simulink model "grid"  (R2025b)
settings: Solver=ode23t  StartTime=0.0  StopTime=0.1  RelTol=1e-3
InitFcn:
  | [P, Q, f_g, f_sw, V_dc, V_g, L_1, L_2, C_f, R_f] = lcl_param();
values from neighbouring files (symbols this model uses):
  f_g = 60    [lcl_param.m]
  f_sw = 5000    [Grid_connected_LCL_filter_code.m]    (also in LCL_filter_code.m; Load_connected_LCL_filter_code.m = 5040; Minor_Final_code.m; lcl_param.m = 15000)
  Q = 250    [lcl_param.m]
  R_f = 3*R_f    [lcl_param.m]
  V_dc = 400    [lcl_param.m]
  V_g = 120 * sqrt(3)    [lcl_param.m]
undefined symbols (not defined in the file or in its folder): PWMGenerator_2_Level__class, Three_PhaseProgrammableV_class, Three_PhaseV_IMeasuremen_class, UniversalBridge_class
libraries: fl_lib x22, nesl_utility x13, ee_lib x5, eeGeneralControl x3, slpidlib x3, eeTransforms x3, eePwmGeneratorTwoLevel x1, eeTotalHarmonicDistorsion x1, sps_lib x1
(part 1 of 2)
settings Model: Creator=swaya  LastModifiedBy=swaya
settings DebuggingCC: SaveWithParameterizedLinksMsg=none

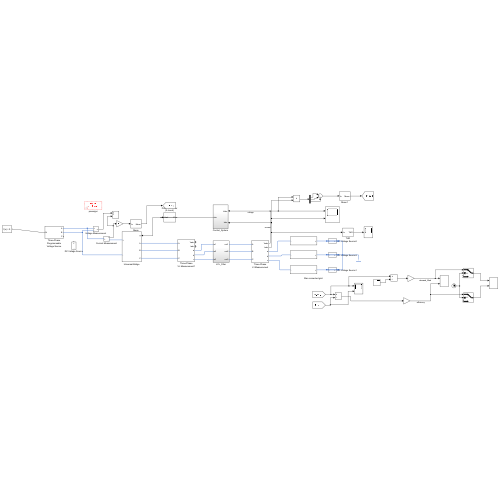
[thumbnail: Simulink's stored preview of the top-level diagram]
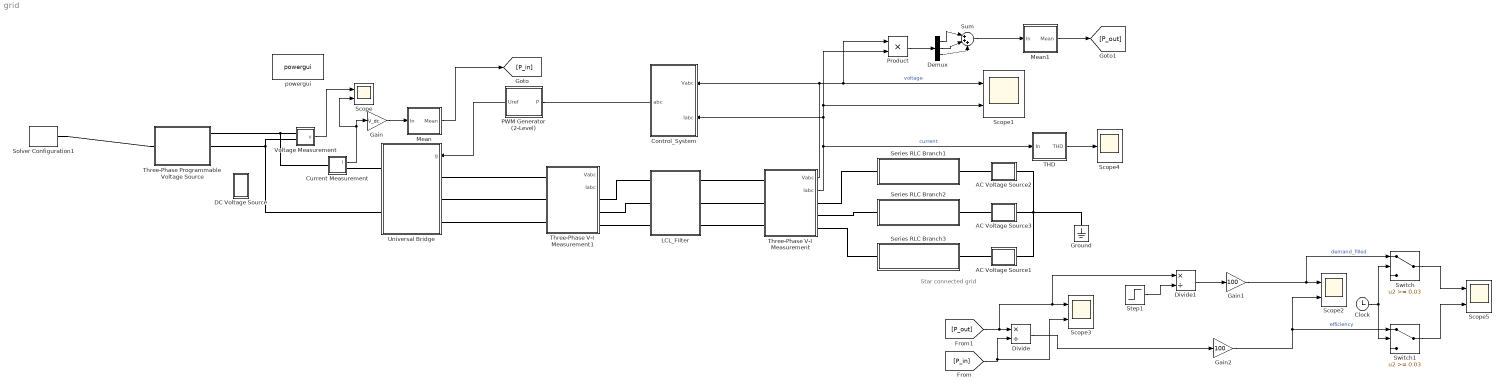
== system grid ==
  note: Star connected grid
  AC Voltage Source1 : Subsystem
      settings: OpenFcn=elec.conv.unmask(gcb);
  AC Voltage Source2 : Subsystem
      settings: OpenFcn=elec.conv.unmask(gcb);
  AC Voltage Source3 : Subsystem
      settings: OpenFcn=elec.conv.unmask(gcb);
  Clock : Clock
  Control_System : Subsystem
  Current Measurement : Subsystem
      settings: OpenFcn=elec.conv.unmask(gcb);
  DC Voltage Source : Subsystem
      settings: OpenFcn=elec.conv.unmask(gcb);
  Demux : Demux  Outputs=3
  Divide : Product  Inputs=*/
  Divide1 : Product  Inputs=*/
  Gain : Gain  Gain=V_dc
  Gain1 : Gain  Gain=100
  Gain2 : Gain  Gain=100
  Ground : fl_lib/Electrical/Electrical Elements/Electrical Reference
  LCL_Filter : Subsystem
  Mean : Subsystem
      settings: OpenFcn=elec.conv.unmask(gcb);
  Mean1 : Subsystem
      settings: OpenFcn=elec.conv.unmask(gcb);
  PWM Generator (2-Level) : Subsystem
      settings: OpenFcn=elec.conv.unmask(gcb);
  Product : Product
  Scope{,1..3,5} (5 alike) : Scope  NumInputPorts=2
      Scope settings: ActiveDisplayYMinimum=387.5  ActiveDisplayYMaximum=512.5
      Scope1 settings: ActiveDisplayYMinimum=-238.93464  ActiveDisplayYMaximum=235.18546  DataLoggingVariableName=ScopeData3
      Scope2 settings: ActiveDisplayYMinimum=-15.53558  ActiveDisplayYMaximum=139.82019  DataLoggingVariableName=ScopeData2
      Scope3 settings: ActiveDisplayYMinimum=-632.55835  ActiveDisplayYMaximum=5693.02515
      Scope5 settings: ActiveDisplayYMinimum=-12.69456  ActiveDisplayYMaximum=114.25108  DataLoggingVariableName=ScopeData4
  Scope4 : Scope
      settings: ActiveDisplayYMinimum=-0.05317  ActiveDisplayYMaximum=0.47849  DataLoggingVariableName=ScopeData3
  Series RLC Branch1 : Subsystem
      settings: OpenFcn=elec.conv.unmask(gcb);
  Series RLC Branch2 : Subsystem
      settings: OpenFcn=elec.conv.unmask(gcb);
  Series RLC Branch3 : Subsystem
      settings: OpenFcn=elec.conv.unmask(gcb);
  Solver Configuration1 : nesl_utility/Solver Configuration  PhysicalDomain=network_engine_domain  SubClassName=solver  LeftPortType=input  RightPortType=generic  Tones=[]  Harmonics=[]  SimulateNoise=off  Profile=off  UseLocalSampling=off  EnableSwitchedLinearOptims=on  FrequencyDomain=off  UseCCode=off  RelTol=0.001  AbsTol=0.001  MinStep=1e-09  ToWorkspace=off  RevertToSquareIcSolve=off  NumHomotopyIterations=100  PhasorMode=off  PhasorModeNumHarmonics=1  ConsistencySolver=NEWTON_XTOL_AFTER_FTOL  IndexReductionMethod=DerivativeReplacement  DoDC=off  ResidualTolerance=1e-09  ConsistencyTolSource=GLOBAL  ConsistencyAbsTol=0.001  ConsistencyRelTol=0.001  ConsistencyTolFactor=0.001  UseLocalSolver=off  LocalSolverChoice=NE_BACKWARD_EULER_ADVANCER  ResolveIndetEquations=on  FunctionEvalNumThread=1  LocalSolverSampleTime=0.001  DoFixedCost=off  MaxNonlinIter=3  MaxModeIter=2  ComputeImpulses=off  ImpulseIterations=2  LinearAlgebra=auto  LinearAlgebraNumThread=0  EquationFormulation=NE_TIME_EF  DelaysMemoryBudget=1024  AutomaticFiltering=on  FilteringTimeConstant=0.001  PartitionStorageMethod=AS_NEEDED  PartitionMemoryBudget=1024  PartitionMethod=ROBUST  MultibodyUseLocalSolver=off  MultibodyLocalSolverChoice=ODE1  MultibodyLocalSolverSampleTime=0.001
  Step1 : Step  Time=0.04  Before=3000  After=5000  SampleTime=0
  Sum : Sum  Inputs=|+++
  Switch : Switch  Threshold=0.03  SaturateOnIntegerOverflow=off  InputSameDT=off
  Switch1 : Switch  Threshold=0.03  SaturateOnIntegerOverflow=off  InputSameDT=off
  THD : Subsystem
      settings: OpenFcn=elec.conv.unmask(gcb);
  Three-Phase Programmable Voltage Source : Subsystem
      settings: OpenFcn=elec.conv.unmask(gcb);
  Three-Phase V-I Measurement : Subsystem
      settings: OpenFcn=elec.conv.unmask(gcb);
  Three-Phase V-I Measurement1 : Subsystem
      settings: OpenFcn=elec.conv.unmask(gcb);
  Universal Bridge : Subsystem
      settings: OpenFcn=elec.conv.unmask(gcb);
  Voltage Measurement : Subsystem
      settings: OpenFcn=elec.conv.unmask(gcb);
  powergui : sps_lib/powergui  Priority=1  SimulationMode=Discrete  SampleTime=50e-8  frequency=60  Iterations=50  frequencyindice=0  Pbase=100e6  ErrMax=1e-4  UnitsV=kV  UnitsW=MW  buscounter=0  FunctionMessages=off  echomessages=off  EnableUseOfTLC=off  CurrentSourceSwitches=off  DisableSnubberDevices=off  DisableRonSwitches=off  DisableVfSwitches=off  DisplayEquations=off  AutomaticDiscreteSolvers=off  SolverType=Tustin/Backward Euler (TBE)  Interpol=off  ExternalGateDelay=off  methode=off  Ts=100  x0status=blocks  SPID=on  SwTol=0  HookPort=off  NonlinearTolerance=1e-4  nMaxIteration=100  ContinueOnMaxIteration=off  RestoreLinks=warning  ResistiveCurrentMeasurement=off  Frange=[0:2:500]  Ylog=off  Xlog=on  ShowGrid=off  save=off  variable=ZData  structure=0  ZoomFFT=off  StartTime=0.0  cycles=1  DisplayStyle=1  fundamental=60  FreqAxis=off  MaxFrequency=1000  frequencyindicesteady=1  RmsSteady=1  display=off
  wires:
  PWM Generator (2-Level)/1(P) -> Universal Bridge/1(g)
  Three-Phase V-I Measurement/1(Vabc) -> Product/1, Scope1/1, Control_System/1(Vabc)  "voltage"
  Three-Phase V-I Measurement/2(Iabc) -> THD/1(In), Product/2, Scope1/2, Control_System/2(Iabc)  "current"
  Control_System/1(abc) -> PWM Generator (2-Level)/1(Uref)
  Product/1 -> Demux/1
  Demux/1 -> Sum/1
  Demux/2 -> Sum/2
  Demux/3 -> Sum/3
  Current Measurement/1(i) -> Scope/2, Gain/1
  THD/1(THD) -> Scope4/1
  Gain/1 -> Mean/1(In)
  [P_out] -> Divide1/1, Scope3/1, Divide/1
  [P_in] -> Scope3/2, Divide/2
  Divide1/1 -> Gain1/1
  Gain1/1 -> Switch/1, Scope2/1  "demand_filled"
  Mean/1(Mean) -> [P_in]
  Divide/1 -> Gain2/1
  Gain2/1 -> Switch1/1, Scope2/2  "efficiency"
  Sum/1 -> Mean1/1(In)
  Mean1/1(Mean) -> [P_out]
  Clock/1 -> Switch/2, Switch1/2
  Switch/1 -> Scope5/1
  Switch1/1 -> Scope5/2
  Step1/1 -> Divide1/2
  Voltage Measurement/1(v) -> Scope/1
  connections:
  LCL_Filter/RConn1 -- Three-Phase V-I Measurement/LConn1
  LCL_Filter/RConn2 -- Three-Phase V-I Measurement/LConn2
  LCL_Filter/RConn3 -- Three-Phase V-I Measurement/LConn3
  Three-Phase V-I Measurement1/LConn1 -- Universal Bridge/LConn1
  Three-Phase V-I Measurement1/LConn2 -- Universal Bridge/LConn2
  Three-Phase V-I Measurement1/LConn3 -- Universal Bridge/LConn3
  Three-Phase V-I Measurement1/RConn1 -- LCL_Filter/LConn1
  Three-Phase V-I Measurement1/RConn2 -- LCL_Filter/LConn2
  Three-Phase V-I Measurement1/RConn3 -- LCL_Filter/LConn3
  Series RLC Branch2/LConn1 -- AC Voltage Source3/RConn1
  AC Voltage Source2/RConn1 -- Series RLC Branch1/LConn1
  Series RLC Branch3/LConn1 -- AC Voltage Source1/RConn1
  AC Voltage Source2/LConn1 -- Ground/LConn1 -- AC Voltage Source1/LConn1 -- AC Voltage Source3/LConn1
  Three-Phase V-I Measurement/RConn1 -- Series RLC Branch1/RConn1
  Three-Phase V-I Measurement/RConn2 -- Series RLC Branch2/RConn1
  Three-Phase V-I Measurement/RConn3 -- Series RLC Branch3/RConn1
  Current Measurement/RConn1 -- Universal Bridge/RConn1
  Three-Phase Programmable Voltage Source/RConn1 -- Current Measurement/LConn1 -- Voltage Measurement/LConn1
  Three-Phase Programmable Voltage Source/RConn2 -- Voltage Measurement/LConn2 -- Universal Bridge/RConn2
  Solver Configuration1/RConn1 -- Three-Phase Programmable Voltage Source/LConn1

== system grid/AC Voltage Source1 ==
  AC Voltage Source : fl_lib/Electrical/Electrical Sources/AC Voltage Source  amp=V_g*sqrt(2/3) V  shift=120 deg  frequency=f_g Hz
  - : PMIOPort  Side=Left
  + : PMIOPort  Port=2  Side=Right
  connections:
  AC Voltage Source/LConn1 -- +/RConn1
  -/RConn1 -- AC Voltage Source/RConn1

== system grid/AC Voltage Source2 ==
  AC Voltage Source : fl_lib/Electrical/Electrical Sources/AC Voltage Source  amp=V_g*sqrt(2/3) V  shift=0 deg  frequency=f_g Hz
  - : PMIOPort  Side=Left
  + : PMIOPort  Port=2  Side=Right
  connections:
  AC Voltage Source/LConn1 -- +/RConn1
  -/RConn1 -- AC Voltage Source/RConn1

== system grid/AC Voltage Source3 ==
  AC Voltage Source : fl_lib/Electrical/Electrical Sources/AC Voltage Source  amp=V_g*sqrt(2/3) V  shift=-120 deg  frequency=f_g Hz
  - : PMIOPort  Side=Left
  + : PMIOPort  Port=2  Side=Right
  connections:
  AC Voltage Source/LConn1 -- +/RConn1
  -/RConn1 -- AC Voltage Source/RConn1

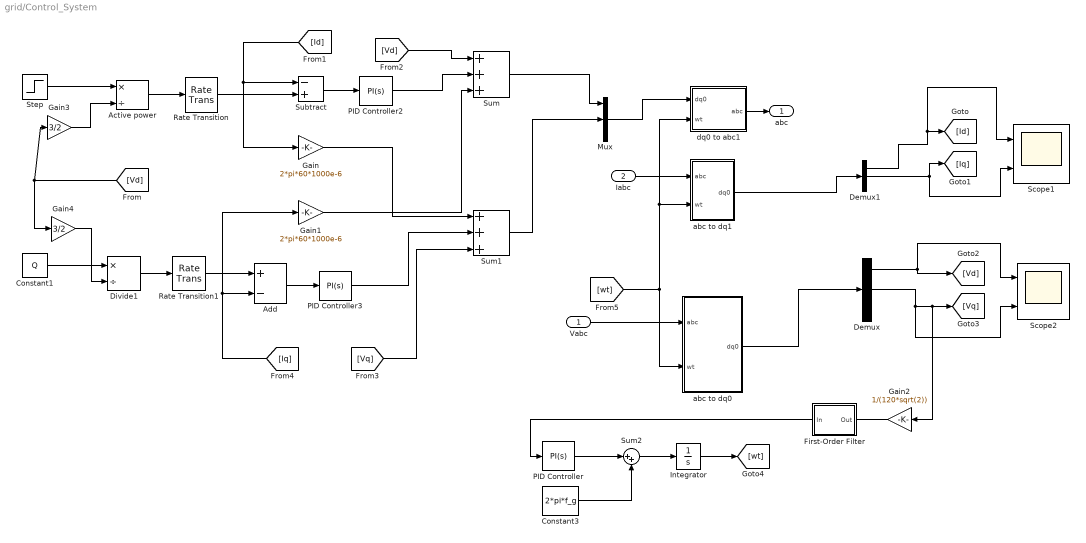
== system grid/Control_System ==
  Vabc : Inport
  Iabc : Inport  Port=2
  Active power : Product  Inputs=*/
  Add : Sum  Inputs=+-
  Constant1 : Constant  Value=Q
  Constant3 : Constant  Value=2*pi*f_g
  Demux : Demux  Outputs=3
  Demux1 : Demux  Outputs=3
  Divide1 : Product  Inputs=*/
  First-Order Filter : Subsystem
      settings: OpenFcn=elec.conv.unmask(gcb);
  Gain : Gain  Gain=2*pi*60*1000e-6
  Gain1 : Gain  Gain=2*pi*60*1000e-6
  Gain2 : Gain  Gain=1/(120*sqrt(2))
  Gain3 : Gain  Gain=3/2
  Gain4 : Gain  Gain=3/2
  Integrator : Integrator
  Mux : Mux  Inputs=3
  PID Controller : slpidlib/PID Controller  Controller=PI  Form=Parallel  TimeDomain=Continuous-time  UseExternalTs=off  SampleTime=-1  IntegratorMethod=Forward Euler  FilterMethod=Forward Euler  ControllerParametersSource=internal  P=-0.26  I=-5.8  UseKiTs=off  D=10  UseExternalDerivativeSource=off  N=100  UseFilter=on  TunerSelectOption=Transfer Function Based (PID Tuner App)  InitialConditionSource=internal  InitialConditionForIntegrator=0  InitialConditionForFilter=0  DifferentiatorICPrevScaledInput=0  ExternalReset=none  TrackingMode=off  Kt=1  LimitOutput=on  SatLimitsSource=internal  UpperSaturationLimit=inf  LowerSaturationLimit=-inf  LinearizeAsGain=on  AntiWindupMode=back-calculation  Kb=1  LimitIntegrator=off  UpperIntegratorSaturationLimit=100  LowerIntegratorSaturationLimit=-inf  POutMin=[]  POutMax=[]  IOutMin=[]  IOutMax=[]  DOutMin=[]  DOutMax=[]  NOutMin=[]  NOutMax=[]  SumOutMin=[]  SumOutMax=[]  SaturationOutMin=[]  SaturationOutMax=[]  PParamMin=[]  PParamMax=[]  IParamMin=[]  IParamMax=[]  DParamMin=[]  DParamMax=[]  NParamMin=[]  NParamMax=[]  KbParamMin=[]  KbParamMax=[]  KtParamMin=[]  KtParamMax=[]  KbOutMin=[]  KbOutMax=[]  KtOutMin=[]  KtOutMax=[]  IntegratorOutMin=[]  IntegratorOutMax=[]  FilterOutMin=[]  FilterOutMax=[]  SumI1OutMin=[]  SumI1OutMax=[]  SumI2OutMin=[]  SumI2OutMax=[]  SumI3OutMin=[]  SumI3OutMax=[]  SumI4OutMin=[]  SumI4OutMax=[]  SumDOutMin=[]  SumDOutMax=[]  DifferentiatorOutMin=[]  DifferentiatorOutMax=[]  FilterDiffOutCoefMin=[]  FilterDiffOutCoefMax=[]  ReciprocalOutMin=[]  ReciprocalOutMax=[]  SumDenOutMin=[]  SumDenOutMax=[]  SumNumOutMin=[]  SumNumOutMax=[]  DivideOutMin=[]  DivideOutMax=[]  UdiffTsProdOutMin=[]  UdiffTsProdOutMax=[]  NTsProdOutMin=[]  NTsProdOutMax=[]  UintegralTsProdOutMin=[]  UintegralTsProdOutMax=[]  UngainTsProdOutMin=[]  UngainTsProdOutMax=[]  ClampingZeroOutDataTypeStr=Inherit: Inherit via back propagation  ClampingZeroOutMin=[]  ClampingZeroOutMax=[]  FilterDenConstantOutDataTypeStr=Inherit: Inherit via back propagation  FilterDenConstantOutMin=[]  FilterDenConstantOutMax=[]  PCopyOutDataTypeStr=Inherit: Inherit via back propagation  PCopyOutMin=[]  PCopyOutMax=[]  NCopyOutDataTypeStr=Inherit: Inherit via back propagation  NCopyOutMin=[]  NCopyOutMax=[]  IntegratorContinuousStateAttributes=''  IntegratorStateMustResolveToSignalObject=off  IntegratorRTWStateStorageClass=Auto  FilterContinuousStateAttributes=''  FilterStateMustResolveToSignalObject=off  FilterRTWStateStorageClass=Auto  ParallelPVariant=InternalParameters  IdealPVariant=Disabled  IVariant=InternalParameters  DVariant=Disabled  IntegratorVariant=Continuous  SatVariant=Enabled  AWVariant=BackCalculation  PCopyVariant=Disabled  TRVariant=Disabled  FdbkBlocksVariant=Forward  IdealPFdbkVariant=Disabled  SatFdbkVariant=Disabled  DerivativeFilterVariant=Disabled  NVariant=Disabled  NCopyVariant=Disabled_SignalSpec  FilterICVariant=Disabled  IntegratorICVariant=InternalICs  ExternalResetVariant=Disabled  TRSumVariant=Passthrough  SumFdbkVariant=Disabled  SumVariant=Sum_PI  TsampFilterVariant=InternalTs  TsampNgainVariant=Passthrough  TsampIntegralVariant=Disabled_SignalSpec  ExternalSaturationOutDataTypeStr=Inherit: Same as second input  DerivativeSourceVariant=Disabled  PreIntVariant=InternalPreInt
  PID Controller2 : slpidlib/PID Controller  Controller=PI  Form=Parallel  TimeDomain=Continuous-time  UseExternalTs=off  SampleTime=-1  IntegratorMethod=Forward Euler  FilterMethod=Forward Euler  ControllerParametersSource=internal  P=5  I=5000  UseKiTs=off  D=5  UseExternalDerivativeSource=off  N=100  UseFilter=on  TunerSelectOption=Transfer Function Based (PID Tuner App)  InitialConditionSource=internal  InitialConditionForIntegrator=0  InitialConditionForFilter=0  DifferentiatorICPrevScaledInput=0  ExternalReset=none  TrackingMode=off  Kt=1  LimitOutput=on  SatLimitsSource=internal  UpperSaturationLimit=inf  LowerSaturationLimit=-inf  LinearizeAsGain=on  AntiWindupMode=back-calculation  Kb=1  LimitIntegrator=off  UpperIntegratorSaturationLimit=inf  LowerIntegratorSaturationLimit=-inf  POutMin=[]  POutMax=[]  IOutMin=[]  IOutMax=[]  DOutMin=[]  DOutMax=[]  NOutMin=[]  NOutMax=[]  SumOutMin=[]  SumOutMax=[]  SaturationOutMin=[]  SaturationOutMax=[]  PParamMin=[]  PParamMax=[]  IParamMin=[]  IParamMax=[]  DParamMin=[]  DParamMax=[]  NParamMin=[]  NParamMax=[]  KbParamMin=[]  KbParamMax=[]  KtParamMin=[]  KtParamMax=[]  KbOutMin=[]  KbOutMax=[]  KtOutMin=[]  KtOutMax=[]  IntegratorOutMin=[]  IntegratorOutMax=[]  FilterOutMin=[]  FilterOutMax=[]  SumI1OutMin=[]  SumI1OutMax=[]  SumI2OutMin=[]  SumI2OutMax=[]  SumI3OutMin=[]  SumI3OutMax=[]  SumI4OutMin=[]  SumI4OutMax=[]  SumDOutMin=[]  SumDOutMax=[]  DifferentiatorOutMin=[]  DifferentiatorOutMax=[]  FilterDiffOutCoefMin=[]  FilterDiffOutCoefMax=[]  ReciprocalOutMin=[]  ReciprocalOutMax=[]  SumDenOutMin=[]  SumDenOutMax=[]  SumNumOutMin=[]  SumNumOutMax=[]  DivideOutMin=[]  DivideOutMax=[]  UdiffTsProdOutMin=[]  UdiffTsProdOutMax=[]  NTsProdOutMin=[]  NTsProdOutMax=[]  UintegralTsProdOutMin=[]  UintegralTsProdOutMax=[]  UngainTsProdOutMin=[]  UngainTsProdOutMax=[]  ClampingZeroOutDataTypeStr=Inherit: Inherit via back propagation  ClampingZeroOutMin=[]  ClampingZeroOutMax=[]  FilterDenConstantOutDataTypeStr=Inherit: Inherit via back propagation  FilterDenConstantOutMin=[]  FilterDenConstantOutMax=[]  PCopyOutDataTypeStr=Inherit: Inherit via back propagation  PCopyOutMin=[]  PCopyOutMax=[]  NCopyOutDataTypeStr=Inherit: Inherit via back propagation  NCopyOutMin=[]  NCopyOutMax=[]  IntegratorContinuousStateAttributes=''  IntegratorStateMustResolveToSignalObject=off  IntegratorRTWStateStorageClass=Auto  FilterContinuousStateAttributes=''  FilterStateMustResolveToSignalObject=off  FilterRTWStateStorageClass=Auto  ParallelPVariant=InternalParameters  IdealPVariant=Disabled  IVariant=InternalParameters  DVariant=Disabled  IntegratorVariant=Continuous  SatVariant=Enabled  AWVariant=BackCalculation  PCopyVariant=Disabled  TRVariant=Disabled  FdbkBlocksVariant=Forward  IdealPFdbkVariant=Disabled  SatFdbkVariant=Disabled  DerivativeFilterVariant=Disabled  NVariant=Disabled  NCopyVariant=Disabled_SignalSpec  FilterICVariant=Disabled  IntegratorICVariant=InternalICs  ExternalResetVariant=Disabled  TRSumVariant=Passthrough  SumFdbkVariant=Disabled  SumVariant=Sum_PI  TsampFilterVariant=InternalTs  TsampNgainVariant=Passthrough  TsampIntegralVariant=Disabled_SignalSpec  ExternalSaturationOutDataTypeStr=Inherit: Same as second input  DerivativeSourceVariant=Disabled  PreIntVariant=InternalPreInt
  PID Controller3 : slpidlib/PID Controller  Controller=PI  Form=Parallel  TimeDomain=Continuous-time  UseExternalTs=off  SampleTime=-1  IntegratorMethod=Forward Euler  FilterMethod=Forward Euler  ControllerParametersSource=internal  P=5  I=5000  UseKiTs=off  D=5  UseExternalDerivativeSource=off  N=100  UseFilter=on  TunerSelectOption=Transfer Function Based (PID Tuner App)  InitialConditionSource=internal  InitialConditionForIntegrator=0  InitialConditionForFilter=0  DifferentiatorICPrevScaledInput=0  ExternalReset=none  TrackingMode=off  Kt=1  LimitOutput=on  SatLimitsSource=internal  UpperSaturationLimit=inf  LowerSaturationLimit=-inf  LinearizeAsGain=on  AntiWindupMode=back-calculation  Kb=1  LimitIntegrator=off  UpperIntegratorSaturationLimit=inf  LowerIntegratorSaturationLimit=-inf  POutMin=[]  POutMax=[]  IOutMin=[]  IOutMax=[]  DOutMin=[]  DOutMax=[]  NOutMin=[]  NOutMax=[]  SumOutMin=[]  SumOutMax=[]  SaturationOutMin=[]  SaturationOutMax=[]  PParamMin=[]  PParamMax=[]  IParamMin=[]  IParamMax=[]  DParamMin=[]  DParamMax=[]  NParamMin=[]  NParamMax=[]  KbParamMin=[]  KbParamMax=[]  KtParamMin=[]  KtParamMax=[]  KbOutMin=[]  KbOutMax=[]  KtOutMin=[]  KtOutMax=[]  IntegratorOutMin=[]  IntegratorOutMax=[]  FilterOutMin=[]  FilterOutMax=[]  SumI1OutMin=[]  SumI1OutMax=[]  SumI2OutMin=[]  SumI2OutMax=[]  SumI3OutMin=[]  SumI3OutMax=[]  SumI4OutMin=[]  SumI4OutMax=[]  SumDOutMin=[]  SumDOutMax=[]  DifferentiatorOutMin=[]  DifferentiatorOutMax=[]  FilterDiffOutCoefMin=[]  FilterDiffOutCoefMax=[]  ReciprocalOutMin=[]  ReciprocalOutMax=[]  SumDenOutMin=[]  SumDenOutMax=[]  SumNumOutMin=[]  SumNumOutMax=[]  DivideOutMin=[]  DivideOutMax=[]  UdiffTsProdOutMin=[]  UdiffTsProdOutMax=[]  NTsProdOutMin=[]  NTsProdOutMax=[]  UintegralTsProdOutMin=[]  UintegralTsProdOutMax=[]  UngainTsProdOutMin=[]  UngainTsProdOutMax=[]  ClampingZeroOutDataTypeStr=Inherit: Inherit via back propagation  ClampingZeroOutMin=[]  ClampingZeroOutMax=[]  FilterDenConstantOutDataTypeStr=Inherit: Inherit via back propagation  FilterDenConstantOutMin=[]  FilterDenConstantOutMax=[]  PCopyOutDataTypeStr=Inherit: Inherit via back propagation  PCopyOutMin=[]  PCopyOutMax=[]  NCopyOutDataTypeStr=Inherit: Inherit via back propagation  NCopyOutMin=[]  NCopyOutMax=[]  IntegratorContinuousStateAttributes=''  IntegratorStateMustResolveToSignalObject=off  IntegratorRTWStateStorageClass=Auto  FilterContinuousStateAttributes=''  FilterStateMustResolveToSignalObject=off  FilterRTWStateStorageClass=Auto  ParallelPVariant=InternalParameters  IdealPVariant=Disabled  IVariant=InternalParameters  DVariant=Disabled  IntegratorVariant=Continuous  SatVariant=Enabled  AWVariant=BackCalculation  PCopyVariant=Disabled  TRVariant=Disabled  FdbkBlocksVariant=Forward  IdealPFdbkVariant=Disabled  SatFdbkVariant=Disabled  DerivativeFilterVariant=Disabled  NVariant=Disabled  NCopyVariant=Disabled_SignalSpec  FilterICVariant=Disabled  IntegratorICVariant=InternalICs  ExternalResetVariant=Disabled  TRSumVariant=Passthrough  SumFdbkVariant=Disabled  SumVariant=Sum_PI  TsampFilterVariant=InternalTs  TsampNgainVariant=Passthrough  TsampIntegralVariant=Disabled_SignalSpec  ExternalSaturationOutDataTypeStr=Inherit: Same as second input  DerivativeSourceVariant=Disabled  PreIntVariant=InternalPreInt
  Rate Transition : RateTransition  OutPortSampleTimeOpt=Inherit
  Rate Transition1 : RateTransition  OutPortSampleTimeOpt=Inherit
  Scope1 : Scope  NumInputPorts=2
      settings: ActiveDisplayYMinimum=-14.64317  ActiveDisplayYMaximum=37.77239
  Scope2 : Scope  NumInputPorts=2
      settings: ActiveDisplayYMinimum=165.62316  ActiveDisplayYMaximum=206.32488  DataLoggingVariableName=ScopeData2
  Step : Step  Time=0.04  Before=3000  After=5000  SampleTime=0
  Subtract : Sum  Inputs=-+
  Sum : Sum  Inputs=+++
  Sum1 : Sum  Inputs=+++
  Sum2 : Sum  Inputs=|++
  abc to dq0 : Subsystem
      settings: OpenFcn=elec.conv.unmask(gcb);
  abc to dq1 : Subsystem
      settings: OpenFcn=elec.conv.unmask(gcb);
  dq0 to abc1 : Subsystem
      settings: OpenFcn=elec.conv.unmask(gcb);
  abc : Outport
  wires:
  Demux1/1 -> [Id], Scope1/1
  [Iq] -> Gain1/1, Add/2
  [Vq] -> Sum1/3
  abc to dq1/1(dq0) -> Demux1/1
  Active power/1 -> Rate Transition/1
  dq0 to abc1/1(abc) -> abc/1
  Gain1/1 -> Sum/3
  [Vd] -> Sum/1
  abc to dq0/1(dq0) -> Demux/1
  [Id] -> Gain/1, Subtract/1
  Constant1/1 -> Divide1/1
  Demux/1 -> [Vd], Scope2/1
  Demux1/2 -> Scope1/2, [Iq]
  Mux/1 -> dq0 to abc1/1(dq0)
  Gain/1 -> Sum1/1
  Iabc/1 -> abc to dq1/1(abc)
  Vabc/1 -> abc to dq0/1(abc)
  Sum/1 -> Mux/1
  Sum1/1 -> Mux/2
  Rate Transition/1 -> Subtract/2
  Divide1/1 -> Rate Transition1/1
  Subtract/1 -> PID Controller2/1
  Add/1 -> PID Controller3/1
  PID Controller2/1 -> Sum/2
  PID Controller3/1 -> Sum1/2
  [wt] -> abc to dq0/2(wt), abc to dq1/2(wt), dq0 to abc1/2(wt)
  Demux/2 -> Scope2/2, Gain2/1, [Vq]
  Constant3/1 -> Sum2/2
  PID Controller/1 -> Sum2/1
  Integrator/1 -> [wt]
  First-Order Filter/1(Out) -> PID Controller/1
  Sum2/1 -> Integrator/1
  Gain2/1 -> First-Order Filter/1(In)
  Rate Transition1/1 -> Add/1
  [Vd] -> Gain4/1, Gain3/1
  Gain3/1 -> Active power/2
  Gain4/1 -> Divide1/2
  Step/1 -> Active power/1

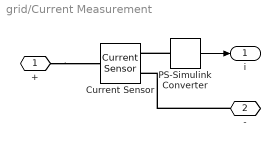
== system grid/Current Measurement ==
  Current Sensor : fl_lib/Electrical/Electrical Sensors/Current Sensor
  PS-Simulink Converter : nesl_utility/PS-Simulink Converter  PhysicalDomain=network_engine_domain  SubClassName=ps_output  LeftPortType=input  RightPortType=output  PseudoPeriodic=off  Frequencies=[]  VectorFormat=1-D array  Unit=A  AffineConversion=off
  + : PMIOPort  Side=Left
  - : PMIOPort  Port=2  Side=Right
  i : Outport  VectorParamsAs1DForOutWhenUnconnected=off
  wires:
  PS-Simulink Converter/1 -> i/1
  connections:
  +/RConn1 -- Current Sensor/LConn1
  -/RConn1 -- Current Sensor/RConn2
  PS-Simulink Converter/LConn1 -- Current Sensor/RConn1

== system grid/DC Voltage Source ==
  DC Voltage Source : fl_lib/Electrical/Electrical Sources/DC Voltage Source  v0=500 V
  - : PMIOPort  Side=Left
  + : PMIOPort  Port=2  Side=Right
  connections:
  DC Voltage Source/RConn1 -- -/RConn1
  DC Voltage Source/LConn1 -- +/RConn1

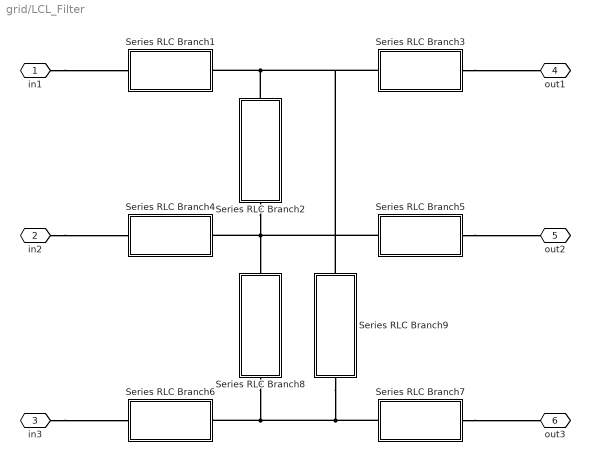
== system grid/LCL_Filter ==
  Series RLC Branch1 : Subsystem
      settings: OpenFcn=elec.conv.unmask(gcb);
  Series RLC Branch2 : Subsystem
      settings: OpenFcn=elec.conv.unmask(gcb);
  Series RLC Branch3 : Subsystem
      settings: OpenFcn=elec.conv.unmask(gcb);
  Series RLC Branch4 : Subsystem
      settings: OpenFcn=elec.conv.unmask(gcb);
  Series RLC Branch5 : Subsystem
      settings: OpenFcn=elec.conv.unmask(gcb);
  Series RLC Branch6 : Subsystem
      settings: OpenFcn=elec.conv.unmask(gcb);
  Series RLC Branch7 : Subsystem
      settings: OpenFcn=elec.conv.unmask(gcb);
  Series RLC Branch8 : Subsystem
      settings: OpenFcn=elec.conv.unmask(gcb);
  Series RLC Branch9 : Subsystem
      settings: OpenFcn=elec.conv.unmask(gcb);
  in1 : PMIOPort  Side=Left
  in2 : PMIOPort  Port=2  Side=Left
  in3 : PMIOPort  Port=3  Side=Left
  out1 : PMIOPort  Port=4  Side=Right
  out2 : PMIOPort  Port=5  Side=Right
  out3 : PMIOPort  Port=6  Side=Right
  connections:
  Series RLC Branch3/LConn1 -- out1/RConn1
  Series RLC Branch2/LConn1 -- Series RLC Branch3/RConn1 -- Series RLC Branch9/LConn1 -- Series RLC Branch1/LConn1
  in1/RConn1 -- Series RLC Branch1/RConn1
  Series RLC Branch5/RConn1 -- Series RLC Branch4/LConn1 -- Series RLC Branch8/LConn1 -- Series RLC Branch2/RConn1
  in2/RConn1 -- Series RLC Branch4/RConn1
  Series RLC Branch5/LConn1 -- out2/RConn1
  Series RLC Branch7/RConn1 -- Series RLC Branch9/RConn1 -- Series RLC Branch6/LConn1 -- Series RLC Branch8/RConn1
  Series RLC Branch7/LConn1 -- out3/RConn1
  in3/RConn1 -- Series RLC Branch6/RConn1

== system grid/Mean ==
  In : Inport
  Moving Average : eeGeneralControl/Moving Average  VariantControl=Variant1  LabelModeActiveChoice=Discrete  f=60  x0=0  BufferSize=8192  Ts=0
  Mean : Outport  VectorParamsAs1DForOutWhenUnconnected=off
  wires:
  Moving Average/1 -> Mean/1
  In/1 -> Moving Average/1

== system grid/Mean1 ==
  In : Inport
  Moving Average : eeGeneralControl/Moving Average  VariantControl=Variant1  LabelModeActiveChoice=Discrete  f=60  x0=0  BufferSize=8192  Ts=0
  Mean : Outport  VectorParamsAs1DForOutWhenUnconnected=off
  wires:
  Moving Average/1 -> Mean/1
  In/1 -> Moving Average/1

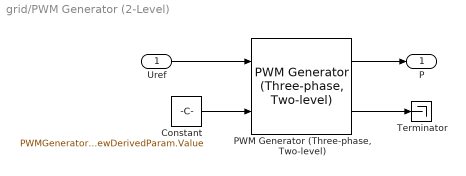
== system grid/PWM Generator (2-Level) ==
  Uref : Inport  SampleTime=PWMGenerator_2_Level__class([-1 1],0,60,f_sw,0,'Three-phase bridge (6 pulses)',0,'Natural').objParamMappingDerived.NewDerivedParam.SampleTime
  Constant : Constant  Value=PWMGenerator_2_Level__class([-1 1],0,60,f_sw,0,'Three-phase bridge (6 pulses)',0,'Natural').objParamMappingDerived.NewDerivedParam.Value  SampleTime=PWMGenerator_2_Level__class([-1 1],0,60,f_sw,0,'Three-phase bridge (6 pulses)',0,'Natural').objParamMappingDerived.NewDerivedParam.SampleTime
  "PWM Generator (Three-phase, Two-level)" : eePwmGeneratorTwoLevel/PWM Generator (Three-phase, Two-level)  PWMMode=Continuous PWM (CPWM)  CPWMMode=SPWM: sinusoidal PWM  DPWMMode=60 DPWM: 60 degree discontinuous PWM  fsw=f_sw  Ts=PWMGenerator_2_Level__class([-1 1],0,60,f_sw,0,'Three-phase bridge (6 pulses)',0,'Natural').objParamMappingDerived.NewDerivedParam.SampleTime
  Terminator : Terminator
  P : Outport  SampleTime=PWMGenerator_2_Level__class([-1 1],0,60,f_sw,0,'Three-phase bridge (6 pulses)',0,'Natural').objParamMappingDerived.NewDerivedParam.SampleTime  VectorParamsAs1DForOutWhenUnconnected=off
  wires:
  "PWM Generator (Three-phase, Two-level)"/2 -> Terminator/1
  "PWM Generator (Three-phase, Two-level)"/1 -> P/1
  Constant/1 -> "PWM Generator (Three-phase, Two-level)"/2
  Uref/1 -> "PWM Generator (Three-phase, Two-level)"/1

== system grid/Series RLC Branch1 ==
  Resistor : fl_lib/Electrical/Electrical Elements/Resistor  R=1 Ohm  i_specify=off  i_priority=None  i=0 A  i_nominal_specify=off  i_nominal_value=1  i_nominal_unit=A  v_specify=off  v_priority=None  v=0 V  v_nominal_specify=off  v_nominal_value=1  v_nominal_unit=V
  + : PMIOPort  Side=Left
  - : PMIOPort  Port=2  Side=Right
  connections:
  +/RConn1 -- Resistor/LConn1
  -/RConn1 -- Resistor/RConn1

== system grid/Series RLC Branch2 ==
  Resistor : fl_lib/Electrical/Electrical Elements/Resistor  R=1 Ohm  i_specify=off  i_priority=None  i=0 A  i_nominal_specify=off  i_nominal_value=1  i_nominal_unit=A  v_specify=off  v_priority=None  v=0 V  v_nominal_specify=off  v_nominal_value=1  v_nominal_unit=V
  + : PMIOPort  Side=Left
  - : PMIOPort  Port=2  Side=Right
  connections:
  +/RConn1 -- Resistor/LConn1
  -/RConn1 -- Resistor/RConn1

== system grid/Series RLC Branch3 ==
  Resistor : fl_lib/Electrical/Electrical Elements/Resistor  R=1 Ohm  i_specify=off  i_priority=None  i=0 A  i_nominal_specify=off  i_nominal_value=1  i_nominal_unit=A  v_specify=off  v_priority=None  v=0 V  v_nominal_specify=off  v_nominal_value=1  v_nominal_unit=V
  + : PMIOPort  Side=Left
  - : PMIOPort  Port=2  Side=Right
  connections:
  +/RConn1 -- Resistor/LConn1
  -/RConn1 -- Resistor/RConn1

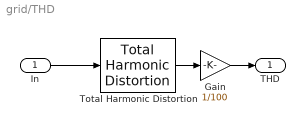
== system grid/THD ==
  In : Inport
  Gain : Gain  Gain=1/100  SampleTime=0
  Total Harmonic Distortion : eeTotalHarmonicDistorsion/Total Harmonic Distortion  f=f_g  Ts=0
  THD : Outport  VectorParamsAs1DForOutWhenUnconnected=off
  wires:
  Gain/1 -> THD/1
  In/1 -> Total Harmonic Distortion/1
  Total Harmonic Distortion/1 -> Gain/1

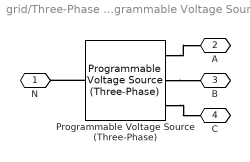
== system grid/Three-Phase Programmable Voltage Source ==
  Programmable Voltage Source (Three-Phase) : ee_lib/Sources/Programmable Voltage Source (Three-Phase)  magnitude_type=3  vline_rms=565.6854 V  magn_ramp=Three_PhaseProgrammableV_class([565.685424949238 0 0],0.25,10,0.3,[3 0.2 -25 0],[2 0.15 35 2]).objParamMappingDerived.NewDerivedParam.magn_ramp V/s  magn_step=Three_PhaseProgrammableV_class([565.685424949238 0 0],0.25,10,0.3,[3 0.2 -25 0],[2 0.15 35 2]).objParamMappingDerived.NewDerivedParam.magn_step V  magn_modu_magn=Three_PhaseProgrammableV_class([565.685424949238 0 0],0.25,10,0.3,[3 0.2 -25 0],[2 0.15 35 2]).objParamMappingDerived.NewDerivedParam.magn_modu_magn V  magn_modu_freq=2 Hz  magn_t1=0.08 s  magn_t2=0.2 s  frequency_type=1  freq=0 Hz  freq_ramp=10 Hz/s  freq_step=0.25 Hz  freq_modu_magn=0.3 Hz  freq_modu_freq=2 Hz  freq_t1=0.08 s  freq_t2=0.2 s  phase_type=1  shift=0 deg  phase_ramp=10 deg/s  phase_step=0.25 deg  phase_modu_magn=0.3 deg  phase_modu_freq=2 Hz  phase_t1=0.08 s  phase_t2=0.2 s  impedance_option=0  SShortCircuit=1e6 V*A  XR=15  R=0.01 Ohm  L=3.97e-4 H  G_parasitic=0 1/Ohm  harmonic_option=0  harmonic_orders=Three_PhaseProgrammableV_class([565.685424949238 0 0],0.25,10,0.3,[3 0.2 -25 0],[2 0.15 35 2]).objParamMappingDerived.NewDerivedParam.harmonic_orders  harmonic_ratios=Three_PhaseProgrammableV_class([565.685424949238 0 0],0.25,10,0.3,[3 0.2 -25 0],[2 0.15 35 2]).objParamMappingDerived.NewDerivedParam.harmonic_ratios  harmonic_shifts=Three_PhaseProgrammableV_class([565.685424949238 0 0],0.25,10,0.3,[3 0.2 -25 0],[2 0.15 35 2]).objParamMappingDerived.NewDerivedParam.harmonic_shifts deg  harmonic_sequences=Three_PhaseProgrammableV_class([565.685424949238 0 0],0.25,10,0.3,[3 0.2 -25 0],[2 0.15 35 2]).objParamMappingDerived.NewDerivedParam.harmonic_sequences  harmonic_t1=0.05 s  harmonic_t2=3 s  I_specify=off  I_priority=None  I=[ 0 0 0 ] A  I_nominal_specify=off  I_nominal_value=1  I_nominal_unit=A  V_specify=off  V_priority=None  V=[ 0 0 0 ] V  V_nominal_specify=off  V_nominal_value=1  V_nominal_unit=V
      settings: InternalSimscapePortConfiguration="{\"Bottom\":[],\"Left\":[{\"id\":\"n\",\"label\":\"n\",\"type\":\"foundation.electrical.electrical\"}],\"Right\":[{\"id\":\"a\",\"label\":\"a\",\"type\":\"foundation.electrical.electrical\"},{\"id\":\"b\",\"label\":\"b\",\"type\":\"foundation.electrical.electrical\"},{\"id\":\"c\",\"label\":\"c\",\"type\":\"foundation.electrical.electrical\"}],\"Top\":[]}"
  N : PMIOPort  Side=Left
  A : PMIOPort  Port=2  Side=Right
  B : PMIOPort  Port=3  Side=Right
  C : PMIOPort  Port=4  Side=Right
  connections:
  Programmable Voltage Source (Three-Phase)/RConn2 -- B/RConn1
  Programmable Voltage Source (Three-Phase)/LConn1 -- N/RConn1
  Programmable Voltage Source (Three-Phase)/RConn3 -- C/RConn1
  Programmable Voltage Source (Three-Phase)/RConn1 -- A/RConn1

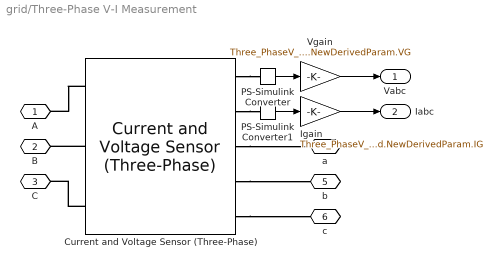
== system grid/Three-Phase V-I Measurement ==
  Current and Voltage Sensor (Three-Phase) : ee_lib/Sensors & Transducers/Current and Voltage Sensor (Three-Phase)  vMeasurementType=2  outputUnit=2  SRated=100000000 V*A  VRated=500000 V  I_specify=off  I_priority=None  I=[ 0 0 0 ] A  I_nominal_specify=off  I_nominal_value=1  I_nominal_unit=A  V_specify=off  V_priority=None  V=[ 0 0 0 ] V  V_nominal_specify=off  V_nominal_value=1  V_nominal_unit=V
      settings: InternalSimscapePortConfiguration="{\"Bottom\":[],\"Left\":[{\"id\":\"a1\",\"label\":\"a1\",\"type\":\"foundation.electrical.electrical\"},{\"id\":\"b1\",\"label\":\"b1\",\"type\":\"foundation.electrical.electrical\"},{\"id\":\"c1\",\"label\":\"c1\",\"type\":\"foundation.electrical.electrical\"}],\"Right\":[{\"id\":\"V_output\",\"label\":\"V\",\"type\":\"output\"},{\"id\":\"I_output\",\"label\":\"I\",\"type\":\"output\"},{\"id\":\"a2\",\"label\":\"a2\",\"type\":\"foundation.electrical.electrical\"},{\"id\":\"b2\",\"label\":\"b2\",\"type\":\"foundation.electrical.electrical\"},{\"id\":\"c2\",\"label\":\"c2\",\"type\":\"foundation.electrical.electrical\"}],\"Top\":[]}"
  Igain : Gain  Gain=Three_PhaseV_IMeasuremen_class('phase-to-ground','yes','off','off','off',100000000,500000).objParamMappingDerived.NewDerivedParam.IG
  PS-Simulink Converter : nesl_utility/PS-Simulink Converter  PhysicalDomain=network_engine_domain  SubClassName=ps_output  LeftPortType=input  RightPortType=output  PseudoPeriodic=off  Frequencies=[]  VectorFormat=1-D array  Unit=1  AffineConversion=off
  PS-Simulink Converter1 : nesl_utility/PS-Simulink Converter  PhysicalDomain=network_engine_domain  SubClassName=ps_output  LeftPortType=input  RightPortType=output  PseudoPeriodic=off  Frequencies=[]  VectorFormat=1-D array  Unit=1  AffineConversion=off
  Vgain : Gain  Gain=Three_PhaseV_IMeasuremen_class('phase-to-ground','yes','off','off','off',100000000,500000).objParamMappingDerived.NewDerivedParam.VG
  A : PMIOPort  Side=Left
  B : PMIOPort  Port=2  Side=Left
  C : PMIOPort  Port=3  Side=Left
  a : PMIOPort  Port=4  Side=Right
  b : PMIOPort  Port=5  Side=Right
  c : PMIOPort  Port=6  Side=Right
  Vabc : Outport  VectorParamsAs1DForOutWhenUnconnected=off
  Iabc : Outport  Port=2  VectorParamsAs1DForOutWhenUnconnected=off
  wires:
  Igain/1 -> Iabc/1
  Vgain/1 -> Vabc/1
  PS-Simulink Converter1/1 -> Igain/1
  PS-Simulink Converter/1 -> Vgain/1
  connections:
  Current and Voltage Sensor (Three-Phase)/RConn1 -- PS-Simulink Converter/LConn1
  Current and Voltage Sensor (Three-Phase)/RConn2 -- PS-Simulink Converter1/LConn1
  Current and Voltage Sensor (Three-Phase)/RConn5 -- c/RConn1
  Current and Voltage Sensor (Three-Phase)/RConn4 -- b/RConn1
  Current and Voltage Sensor (Three-Phase)/RConn3 -- a/RConn1
  Current and Voltage Sensor (Three-Phase)/LConn3 -- C/RConn1
  Current and Voltage Sensor (Three-Phase)/LConn1 -- A/RConn1
  Current and Voltage Sensor (Three-Phase)/LConn2 -- B/RConn1

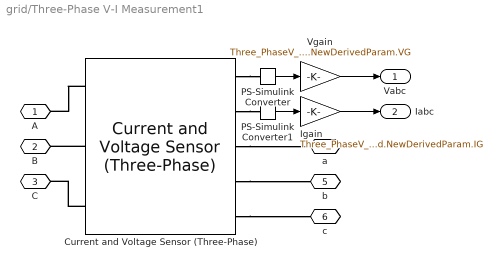
== system grid/Three-Phase V-I Measurement1 ==
  Current and Voltage Sensor (Three-Phase) : ee_lib/Sensors & Transducers/Current and Voltage Sensor (Three-Phase)  vMeasurementType=2  outputUnit=2  SRated=100000000 V*A  VRated=500000 V  I_specify=off  I_priority=None  I=[ 0 0 0 ] A  I_nominal_specify=off  I_nominal_value=1  I_nominal_unit=A  V_specify=off  V_priority=None  V=[ 0 0 0 ] V  V_nominal_specify=off  V_nominal_value=1  V_nominal_unit=V
      settings: InternalSimscapePortConfiguration="{\"Bottom\":[],\"Left\":[{\"id\":\"a1\",\"label\":\"a1\",\"type\":\"foundation.electrical.electrical\"},{\"id\":\"b1\",\"label\":\"b1\",\"type\":\"foundation.electrical.electrical\"},{\"id\":\"c1\",\"label\":\"c1\",\"type\":\"foundation.electrical.electrical\"}],\"Right\":[{\"id\":\"V_output\",\"label\":\"V\",\"type\":\"output\"},{\"id\":\"I_output\",\"label\":\"I\",\"type\":\"output\"},{\"id\":\"a2\",\"label\":\"a2\",\"type\":\"foundation.electrical.electrical\"},{\"id\":\"b2\",\"label\":\"b2\",\"type\":\"foundation.electrical.electrical\"},{\"id\":\"c2\",\"label\":\"c2\",\"type\":\"foundation.electrical.electrical\"}],\"Top\":[]}"
  Igain : Gain  Gain=Three_PhaseV_IMeasuremen_class('phase-to-ground','yes','off','off','off',100000000,500000).objParamMappingDerived.NewDerivedParam.IG
  PS-Simulink Converter : nesl_utility/PS-Simulink Converter  PhysicalDomain=network_engine_domain  SubClassName=ps_output  LeftPortType=input  RightPortType=output  PseudoPeriodic=off  Frequencies=[]  VectorFormat=1-D array  Unit=1  AffineConversion=off
  PS-Simulink Converter1 : nesl_utility/PS-Simulink Converter  PhysicalDomain=network_engine_domain  SubClassName=ps_output  LeftPortType=input  RightPortType=output  PseudoPeriodic=off  Frequencies=[]  VectorFormat=1-D array  Unit=1  AffineConversion=off
  Vgain : Gain  Gain=Three_PhaseV_IMeasuremen_class('phase-to-ground','yes','off','off','off',100000000,500000).objParamMappingDerived.NewDerivedParam.VG
  A : PMIOPort  Side=Left
  B : PMIOPort  Port=2  Side=Left
  C : PMIOPort  Port=3  Side=Left
  a : PMIOPort  Port=4  Side=Right
  b : PMIOPort  Port=5  Side=Right
  c : PMIOPort  Port=6  Side=Right
  Vabc : Outport  VectorParamsAs1DForOutWhenUnconnected=off
  Iabc : Outport  Port=2  VectorParamsAs1DForOutWhenUnconnected=off
  wires:
  Igain/1 -> Iabc/1
  Vgain/1 -> Vabc/1
  PS-Simulink Converter1/1 -> Igain/1
  PS-Simulink Converter/1 -> Vgain/1
  connections:
  Current and Voltage Sensor (Three-Phase)/RConn1 -- PS-Simulink Converter/LConn1
  Current and Voltage Sensor (Three-Phase)/RConn2 -- PS-Simulink Converter1/LConn1
  Current and Voltage Sensor (Three-Phase)/RConn5 -- c/RConn1
  Current and Voltage Sensor (Three-Phase)/RConn4 -- b/RConn1
  Current and Voltage Sensor (Three-Phase)/RConn3 -- a/RConn1
  Current and Voltage Sensor (Three-Phase)/LConn3 -- C/RConn1
  Current and Voltage Sensor (Three-Phase)/LConn1 -- A/RConn1
  Current and Voltage Sensor (Three-Phase)/LConn2 -- B/RConn1

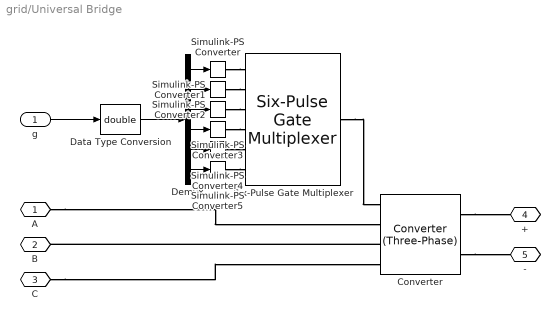
== system grid/Universal Bridge ==
  g : Inport
  Converter : ee_lib/Semiconductors & Converters/Converters/Converter (Three-Phase)  port_option=ee.enum.threePhasePort.expanded  fidelity_option=ee.enum.converters.fidelity.detailed  device_type=3  showThermalPort=false  K=0  Vth=0.5 V  Vgt=0.5 V  Vgt_off=0.1 V  Ih=0.1 A  Vf=UniversalBridge_class('3','IGBT / Diodes',[0 0],0,100000,Inf,0.001).objParamMappingDerived.NewDerivedParam.Vf V  Ron=UniversalBridge_class('3','IGBT / Diodes',[0 0],0,100000,Inf,0.001).objParamMappingDerived.NewDerivedParam.Ron Ohm  Rds=UniversalBridge_class('3','IGBT / Diodes',[0 0],0,100000,Inf,0.001).objParamMappingDerived.NewDerivedParam.Rds Ohm  Goff=UniversalBridge_class('3','IGBT / Diodes',[0 0],0,100000,Inf,0.001).objParamMappingDerived.NewDerivedParam.Goff 1/Ohm  Eon_scalar=22.86e-3 J  Eoff_scalar=17.14e-3 J  Eoff_natural_commutation=10e-3 J  Voff=300 V  Iout_scalar=600 A  onCurrentMeasDelay=0 s  useCurrentFromPreviousCycle=false  useVoltageFromPreviousCycle=false  diode_param=2  diode_Vf=UniversalBridge_class('3','IGBT / Diodes',[0 0],0,100000,Inf,0.001).objParamMappingDerived.NewDerivedParam.diode_Vf V  diode_Ron=UniversalBridge_class('3','IGBT / Diodes',[0 0],0,100000,Inf,0.001).objParamMappingDerived.NewDerivedParam.diode_Ron Ohm  diode_Goff=UniversalBridge_class('3','IGBT / Diodes',[0 0],0,100000,Inf,0.001).objParamMappingDerived.NewDerivedParam.diode_Goff 1/Ohm  diode_C=50 nF  diode_iRM=-235 A  diode_iF=300 A  diode_idot=-50 A/us  diode_trr_param=ee.enum.converters.diodetrr.trr_factor  diode_trr_factor=3  diode_trr=15 us  diode_Qrr=1.5e+3 s*uA  diode_rec_loss_model=ee.enum.diode.reverseRecoveryModel.fixed  diode_ErecVal=0 J  diode_scaleWithIandV=false  diode_ErecMat=zeros(2, 3) J  diode_TjrecVec=[298.15, 398.15] K  diode_IfrecVec=[.1, 1, 10] A  diode_IrecVal=10 A  diode_VrecVal=10 V  diode_tFilter=1 / 1000 / 100 s  thermal_network_parameterization=ee.enum.thermalNetworkTopology.external  Rth=[.08, .5] K/W  Rth_Cauer=[.08, .1, .5] K/W  Rth_Foster=[.08, .14, .22, .16] K/W  thermal_mass_parameterization=ee.enum.thermalNetwork.timeconstant  thermal_mass=[.01, .5] J/K  thermal_mass_Cauer=[.01, .1, .5] J/K  thermal_mass_Foster=[.001, .005, .05, .5] J/K  thermal_time_constant=[.001, .2] s  thermal_time_constant_Cauer=[.001, .1, .2] s  thermal_time_constant_Foster=[7e-05, .0007, .01, .08] s  thermal_mass_initial_temperatures=[25, 25] degC  thermal_mass_initial_temperatures_Cauer=[25, 25, 25] degC  junction_thermal_mass=0.01 J/K  Tvec_initial_Foster=[25, 25, 25, 25] degC  snubber_type=0  Cs=UniversalBridge_class('3','IGBT / Diodes',[0 0],0,100000,Inf,0.001).objParamMappingDerived.NewDerivedParam.Cs F  Rs=UniversalBridge_class('3','IGBT / Diodes',[0 0],0,100000,Inf,0.001).objParamMappingDerived.NewDerivedParam.Rs Ohm  Vce_loss=[0, 150, 300] V
      settings: InternalSimscapePortConfiguration="{\"Bottom\":[],\"Left\":[{\"id\":\"G\",\"label\":\"G\",\"type\":\"foundation.electrical.twelve_phase\"},{\"id\":\"a\",\"label\":\"a\",\"type\":\"foundation.electrical.electrical\"},{\"id\":\"b\",\"label\":\"b\",\"type\":\"foundation.electrical.electrical\"},{\"id\":\"c\",\"label\":\"c\",\"type\":\"foundation.electrical.electrical\"}],\"Right\":[{\"id\":\"p\",\"label\":\"+\",\"type\":\"foundation.electrical.electrical\"},{\"id\":\"n\",\"label\":\"-\",\"type\":\"foundation.electrical.electrical\"}],\"Top\":[]}"
  Data Type Conversion : DataTypeConversion  OutDataTypeStr=double  SaturateOnIntegerOverflow=off  RndMeth=Floor
  Demux : Demux  Outputs=6
  Simulink-PS Converter{,1..5} (6 alike) : nesl_utility/Simulink-PS Converter  PhysicalDomain=network_engine_domain  SubClassName=ps_input  LeftPortType=input  RightPortType=output  PseudoPeriodic=off  Frequencies=[]  NoiseDistribution=none  NoiseParameters=[]  Unit=1  AffineConversion=off  FilteringAndDerivatives=provide  SimscapeFilterOrder=1  InputFilterTimeConstant=0.001  UdotUserProvided=0
  Six-Pulse Gate Multiplexer : ee_lib/Semiconductors & Converters/Converters/Six-Pulse Gate Multiplexer  port_option=ee.enum.controlport.ps
  A : PMIOPort  Side=Left
  B : PMIOPort  Port=2  Side=Left
  C : PMIOPort  Port=3  Side=Left
  + : PMIOPort  Port=4  Side=Right
  - : PMIOPort  Port=5  Side=Right
  wires:
  Data Type Conversion/1 -> Demux/1
  Demux/6 -> Simulink-PS Converter5/1
  Demux/5 -> Simulink-PS Converter4/1
  Demux/4 -> Simulink-PS Converter3/1
  Demux/3 -> Simulink-PS Converter2/1
  Demux/2 -> Simulink-PS Converter1/1
  Demux/1 -> Simulink-PS Converter/1
  g/1 -> Data Type Conversion/1
  connections:
  Converter/RConn2 -- -/RConn1
  Converter/RConn1 -- +/RConn1
  C/RConn1 -- Converter/LConn4
  A/RConn1 -- Converter/LConn2
  Converter/LConn3 -- B/RConn1
  Simulink-PS Converter5/RConn1 -- Six-Pulse Gate Multiplexer/LConn6
  Simulink-PS Converter4/RConn1 -- Six-Pulse Gate Multiplexer/LConn5
  Simulink-PS Converter3/RConn1 -- Six-Pulse Gate Multiplexer/LConn4
  Simulink-PS Converter2/RConn1 -- Six-Pulse Gate Multiplexer/LConn3
  Simulink-PS Converter/RConn1 -- Six-Pulse Gate Multiplexer/LConn1
  Simulink-PS Converter1/RConn1 -- Six-Pulse Gate Multiplexer/LConn2
  Six-Pulse Gate Multiplexer/RConn1 -- Converter/LConn1

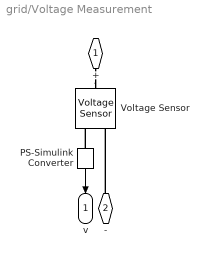
== system grid/Voltage Measurement ==
  PS-Simulink Converter : nesl_utility/PS-Simulink Converter  PhysicalDomain=network_engine_domain  SubClassName=ps_output  LeftPortType=input  RightPortType=output  PseudoPeriodic=off  Frequencies=[]  VectorFormat=1-D array  Unit=V  AffineConversion=off
  Voltage Sensor : fl_lib/Electrical/Electrical Sensors/Voltage Sensor
  + : PMIOPort  Side=Left
  - : PMIOPort  Port=2  Side=Left
  v : Outport  VectorParamsAs1DForOutWhenUnconnected=off
  wires:
  PS-Simulink Converter/1 -> v/1
  connections:
  PS-Simulink Converter/LConn1 -- Voltage Sensor/RConn1
  -/RConn1 -- Voltage Sensor/RConn2
  +/RConn1 -- Voltage Sensor/LConn1

== system grid/Control_System/First-Order Filter ==
  In : Inport
  Low-Pass Filter (Discrete or Continuous) : eeGeneralControl/Low-Pass Filter (Discrete or Continuous)  K=1  T=0.002  B=inf  A=-inf  init_option=Inherited from block input  x0=0  Ts=0
  Out : Outport  VectorParamsAs1DForOutWhenUnconnected=off
  wires:
  Low-Pass Filter (Discrete or Continuous)/1 -> Out/1
  In/1 -> Low-Pass Filter (Discrete or Continuous)/1

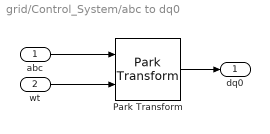
== system grid/Control_System/abc to dq0 ==
  abc : Inport
  wt : Inport  Port=2
  Park Transform : eeTransforms/Park Transform  AxisAlignment=Q-axis  PowerInvariant=off
  dq0 : Outport  VectorParamsAs1DForOutWhenUnconnected=off
  wires:
  Park Transform/1 -> dq0/1
  abc/1 -> Park Transform/1
  wt/1 -> Park Transform/2

== system grid/Control_System/abc to dq1 ==
  abc : Inport
  wt : Inport  Port=2
  Park Transform : eeTransforms/Park Transform  AxisAlignment=Q-axis  PowerInvariant=off
  dq0 : Outport  VectorParamsAs1DForOutWhenUnconnected=off
  wires:
  Park Transform/1 -> dq0/1
  abc/1 -> Park Transform/1
  wt/1 -> Park Transform/2

== system grid/Control_System/dq0 to abc1 ==
  dq0 : Inport
  wt : Inport  Port=2
  Inverse Park Transform : eeTransforms/Inverse Park Transform  AxisAlignment=Q-axis  PowerInvariant=off
  abc : Outport  VectorParamsAs1DForOutWhenUnconnected=off
  wires:
  Inverse Park Transform/1 -> abc/1
  dq0/1 -> Inverse Park Transform/1
  wt/1 -> Inverse Park Transform/2

== system grid/LCL_Filter/Series RLC Branch1 ==
  Inductor : fl_lib/Electrical/Electrical Elements/Inductor  l=L_1 H  r=0 Ohm  g=1e-9 1/Ohm  i_specify=off  i_priority=None  i=0 A  i_nominal_specify=off  i_nominal_value=1  i_nominal_unit=A  v_specify=off  v_priority=None  v=0 V  v_nominal_specify=off  v_nominal_value=1  v_nominal_unit=V  i_L_specify=on  i_L_priority=None  i_L=0 A  i_L_nominal_specify=off  i_L_nominal_value=1  i_L_nominal_unit=A
  + : PMIOPort  Side=Left
  - : PMIOPort  Port=2  Side=Right
  connections:
  -/RConn1 -- Inductor/RConn1
  Inductor/LConn1 -- +/RConn1

== system grid/LCL_Filter/Series RLC Branch2 ==
  Capacitor : fl_lib/Electrical/Electrical Elements/Capacitor  c=C_f F  r=1e-6 Ohm  g=0 1/Ohm  i_specify=off  i_priority=None  i=0 A  i_nominal_specify=off  i_nominal_value=1  i_nominal_unit=A  v_specify=off  v_priority=None  v=0 V  v_nominal_specify=off  v_nominal_value=1  v_nominal_unit=V  vc_specify=on  vc_priority=None  vc=0 V  vc_nominal_specify=off  vc_nominal_value=1  vc_nominal_unit=V
  Resistor : fl_lib/Electrical/Electrical Elements/Resistor  R=R_f Ohm  i_specify=off  i_priority=None  i=0 A  i_nominal_specify=off  i_nominal_value=1  i_nominal_unit=A  v_specify=off  v_priority=None  v=0 V  v_nominal_specify=off  v_nominal_value=1  v_nominal_unit=V
  + : PMIOPort  Side=Left
  - : PMIOPort  Port=2  Side=Right
  connections:
  Capacitor/RConn1 -- -/RConn1
  +/RConn1 -- Resistor/LConn1
  Resistor/RConn1 -- Capacitor/LConn1

== system grid/LCL_Filter/Series RLC Branch3 ==
  Inductor : fl_lib/Electrical/Electrical Elements/Inductor  l=L_2 H  r=0 Ohm  g=1e-9 1/Ohm  i_specify=off  i_priority=None  i=0 A  i_nominal_specify=off  i_nominal_value=1  i_nominal_unit=A  v_specify=off  v_priority=None  v=0 V  v_nominal_specify=off  v_nominal_value=1  v_nominal_unit=V  i_L_specify=on  i_L_priority=None  i_L=0 A  i_L_nominal_specify=off  i_L_nominal_value=1  i_L_nominal_unit=A
  + : PMIOPort  Side=Left
  - : PMIOPort  Port=2  Side=Right
  connections:
  -/RConn1 -- Inductor/RConn1
  Inductor/LConn1 -- +/RConn1

== system grid/LCL_Filter/Series RLC Branch4 ==
  Inductor : fl_lib/Electrical/Electrical Elements/Inductor  l=L_1 H  r=0 Ohm  g=1e-9 1/Ohm  i_specify=off  i_priority=None  i=0 A  i_nominal_specify=off  i_nominal_value=1  i_nominal_unit=A  v_specify=off  v_priority=None  v=0 V  v_nominal_specify=off  v_nominal_value=1  v_nominal_unit=V  i_L_specify=on  i_L_priority=None  i_L=0 A  i_L_nominal_specify=off  i_L_nominal_value=1  i_L_nominal_unit=A
  + : PMIOPort  Side=Left
  - : PMIOPort  Port=2  Side=Right
  connections:
  -/RConn1 -- Inductor/RConn1
  Inductor/LConn1 -- +/RConn1

== system grid/LCL_Filter/Series RLC Branch5 ==
  Inductor : fl_lib/Electrical/Electrical Elements/Inductor  l=L_2 H  r=0 Ohm  g=1e-9 1/Ohm  i_specify=off  i_priority=None  i=0 A  i_nominal_specify=off  i_nominal_value=1  i_nominal_unit=A  v_specify=off  v_priority=None  v=0 V  v_nominal_specify=off  v_nominal_value=1  v_nominal_unit=V  i_L_specify=on  i_L_priority=None  i_L=0 A  i_L_nominal_specify=off  i_L_nominal_value=1  i_L_nominal_unit=A
  + : PMIOPort  Side=Left
  - : PMIOPort  Port=2  Side=Right
  connections:
  -/RConn1 -- Inductor/RConn1
  Inductor/LConn1 -- +/RConn1

== system grid/LCL_Filter/Series RLC Branch6 ==
  Inductor : fl_lib/Electrical/Electrical Elements/Inductor  l=L_1 H  r=0 Ohm  g=1e-9 1/Ohm  i_specify=off  i_priority=None  i=0 A  i_nominal_specify=off  i_nominal_value=1  i_nominal_unit=A  v_specify=off  v_priority=None  v=0 V  v_nominal_specify=off  v_nominal_value=1  v_nominal_unit=V  i_L_specify=on  i_L_priority=None  i_L=0 A  i_L_nominal_specify=off  i_L_nominal_value=1  i_L_nominal_unit=A
  + : PMIOPort  Side=Left
  - : PMIOPort  Port=2  Side=Right
  connections:
  -/RConn1 -- Inductor/RConn1
  Inductor/LConn1 -- +/RConn1

== system grid/LCL_Filter/Series RLC Branch7 ==
  Inductor : fl_lib/Electrical/Electrical Elements/Inductor  l=L_2 H  r=0 Ohm  g=1e-9 1/Ohm  i_specify=off  i_priority=None  i=0 A  i_nominal_specify=off  i_nominal_value=1  i_nominal_unit=A  v_specify=off  v_priority=None  v=0 V  v_nominal_specify=off  v_nominal_value=1  v_nominal_unit=V  i_L_specify=on  i_L_priority=None  i_L=0 A  i_L_nominal_specify=off  i_L_nominal_value=1  i_L_nominal_unit=A
  + : PMIOPort  Side=Left
  - : PMIOPort  Port=2  Side=Right
  connections:
  -/RConn1 -- Inductor/RConn1
  Inductor/LConn1 -- +/RConn1

== system grid/LCL_Filter/Series RLC Branch8 ==
  Capacitor : fl_lib/Electrical/Electrical Elements/Capacitor  c=C_f F  r=1e-6 Ohm  g=0 1/Ohm  i_specify=off  i_priority=None  i=0 A  i_nominal_specify=off  i_nominal_value=1  i_nominal_unit=A  v_specify=off  v_priority=None  v=0 V  v_nominal_specify=off  v_nominal_value=1  v_nominal_unit=V  vc_specify=on  vc_priority=None  vc=0 V  vc_nominal_specify=off  vc_nominal_value=1  vc_nominal_unit=V
  Resistor : fl_lib/Electrical/Electrical Elements/Resistor  R=R_f Ohm  i_specify=off  i_priority=None  i=0 A  i_nominal_specify=off  i_nominal_value=1  i_nominal_unit=A  v_specify=off  v_priority=None  v=0 V  v_nominal_specify=off  v_nominal_value=1  v_nominal_unit=V
  + : PMIOPort  Side=Left
  - : PMIOPort  Port=2  Side=Right
  connections:
  Capacitor/RConn1 -- -/RConn1
  +/RConn1 -- Resistor/LConn1
  Resistor/RConn1 -- Capacitor/LConn1
